simulink model "Candidacy_Exam_RR"  (R2023a)
settings: Solver=VariableStepAuto  StartTime=0  StopTime=1000  FixedStep=0.01  RelTol=1e-3
model workspace (MAT data in the model file):
  finalint = 0
  firstWarning = 1
  originalScenarioChecksum = '114339432DE22364D47BB28FC96DC10C'
undefined symbols (not defined in the file): Acceleration, ActorID, AngularVelocity, curvature, DefaultGear, Defined, DEND_B, DEND_S, DEND_T, direction, DiscIntNeverNeededParam, driving, Ego, EgoRefPose, gradbp, L, Lane, LF, LR, m, matlabshared, MAX_BRAKE, MAX_STEER, MAX_TORQUE, maxNumActors, MCAR, MIN_BRAKE, MIN_STEER, MIN_TORQUE, n, NUMD_B, NUMD_S, NUMD_T, Pitch, Pose, Position, psi_o, R, Roll, RRdamp, SceneInfo, session, sigbuilder_block, STEER_RATIO, stopSign_ID, Tdead, thetaRefs, TL_ID, TrackWidth, Ts, ts, User, Vdead, Velocity, WB, X_o, xRef2s, Y_o, Yaw, yRef2s
libraries: drivingscenarioandsensors x13, roadrunnerscenario x11, simulink x8, simulink_extras x5, drivingvehiclecontroller x2, trackingutilitieslib x2, robotalgslib x1, mpcadaslib x1, slpidlib x1, drivinglib x1, autolibshared x1, vehdynlibviscommon x1
(part 4 of 5)

== system Candidacy_Exam_RR/Reference Data1/Subsystem1/Subsystem3/Subsystem/Theta ==
  note: 1) Add Subsystem or Model blocks as valid variant choices.
      | 2) You cannot connect blocks at this level. At simulation, connectivity is automatically
      | determined, based on the active variant and port name matching.
  y : Inport
  x : Inport  Port=2
  dis : Inport  Port=3
  thetaBlocks : Subsystem  VariantControl=thetaSimulinkBlock
  thetaLt : Subsystem  VariantControl=thetaLookUpTable
  theta : Outport

== system Candidacy_Exam_RR/Reference Data1/Subsystem2/Subsystem/Theta/thetaBlocks ==
  note: theta calculated from Simulink blocks
  y : Inport
  x : Inport  Port=2
  dis : Inport  Port=3
  Atan2 : Trigonometry  Operator=atan2  ApproximationMethod=CORDIC
  Difference : simulink/Discrete/Difference  ICPrevInput=0.0  OutMin=[]  OutMax=[]  OutDataType=fixdt(1, 16)  OutScaling=2^-10  DoSatur=off
  Difference1 : simulink/Discrete/Difference  ICPrevInput=0.0  OutMin=[]  OutMax=[]  OutDataType=fixdt(1, 16)  OutScaling=2^-10  DoSatur=off
  IC : InitialCondition  Value=psi_o
  Radians to Degrees : simulink_extras/Transformations/Radians to Degrees
  Terminator : Terminator
  theta : Outport
  wires:
  IC/1 -> Radians to Degrees/1
  Atan2/1 -> IC/1
  dis/1 -> Terminator/1
  x/1 -> Difference1/1
  y/1 -> Difference/1
  Radians to Degrees/1 -> theta/1
  Difference/1 -> Atan2/1
  Difference1/1 -> Atan2/2

== system Candidacy_Exam_RR/Reference Data1/Subsystem2/Subsystem/Theta/thetaLt ==
  note: Check out the script "setUpModel" to understand how we have calculated theta
  note: theta based on lookup table
  y : Inport
  x : Inport  Port=2
  dis : Inport  Port=3
  Terminator : Terminator
  Terminator1 : Terminator
  Theta Ref : Lookup_n-D  NumberOfTableDimensions=1  BreakpointsForDimension1=gradbp  Table=thetaRefs  InternalRulePriority=Speed  RndMeth=Simplest
  theta : Outport
  wires:
  Theta Ref/1 -> theta/1
  dis/1 -> Theta Ref/1
  x/1 -> Terminator1/1
  y/1 -> Terminator/1

== system Candidacy_Exam_RR/Reference Data1/Subsystem3/Subsystem/Theta/thetaBlocks ==
  note: theta calculated from Simulink blocks
  y : Inport
  x : Inport  Port=2
  dis : Inport  Port=3
  Atan2 : Trigonometry  Operator=atan2  ApproximationMethod=CORDIC
  Difference : simulink/Discrete/Difference  ICPrevInput=0.0  OutMin=[]  OutMax=[]  OutDataType=fixdt(1, 16)  OutScaling=2^-10  DoSatur=off
  Difference1 : simulink/Discrete/Difference  ICPrevInput=0.0  OutMin=[]  OutMax=[]  OutDataType=fixdt(1, 16)  OutScaling=2^-10  DoSatur=off
  IC : InitialCondition  Value=psi_o
  Radians to Degrees : simulink_extras/Transformations/Radians to Degrees
  Terminator : Terminator
  theta : Outport
  wires:
  IC/1 -> Radians to Degrees/1
  Atan2/1 -> IC/1
  dis/1 -> Terminator/1
  x/1 -> Difference1/1
  y/1 -> Difference/1
  Radians to Degrees/1 -> theta/1
  Difference/1 -> Atan2/1
  Difference1/1 -> Atan2/2

== system Candidacy_Exam_RR/Reference Data1/Subsystem3/Subsystem/Theta/thetaLt ==
  note: Check out the script "setUpModel" to understand how we have calculated theta
  note: theta based on lookup table
  y : Inport
  x : Inport  Port=2
  dis : Inport  Port=3
  Terminator : Terminator
  Terminator1 : Terminator
  Theta Ref : Lookup_n-D  NumberOfTableDimensions=1  BreakpointsForDimension1=gradbp  Table=thetaRefs  InternalRulePriority=Speed  RndMeth=Simplest
  theta : Outport
  wires:
  Theta Ref/1 -> theta/1
  dis/1 -> Theta Ref/1
  x/1 -> Terminator1/1
  y/1 -> Terminator/1

== system Candidacy_Exam_RR/Reference Data1/Subsystem1/Subsystem2/Subsystem/Theta/thetaBlocks ==
  note: theta calculated from Simulink blocks
  y : Inport
  x : Inport  Port=2
  dis : Inport  Port=3
  Atan2 : Trigonometry  Operator=atan2  ApproximationMethod=CORDIC
  Difference : simulink/Discrete/Difference  ICPrevInput=0.0  OutMin=[]  OutMax=[]  OutDataType=fixdt(1, 16)  OutScaling=2^-10  DoSatur=off
  Difference1 : simulink/Discrete/Difference  ICPrevInput=0.0  OutMin=[]  OutMax=[]  OutDataType=fixdt(1, 16)  OutScaling=2^-10  DoSatur=off
  IC : InitialCondition  Value=psi_o
  Radians to Degrees : simulink_extras/Transformations/Radians to Degrees
  Terminator : Terminator
  theta : Outport
  wires:
  IC/1 -> Radians to Degrees/1
  Atan2/1 -> IC/1
  dis/1 -> Terminator/1
  x/1 -> Difference1/1
  y/1 -> Difference/1
  Radians to Degrees/1 -> theta/1
  Difference/1 -> Atan2/1
  Difference1/1 -> Atan2/2

== system Candidacy_Exam_RR/Reference Data1/Subsystem1/Subsystem2/Subsystem/Theta/thetaLt ==
  note: Check out the script "setUpModel" to understand how we have calculated theta
  note: theta based on lookup table
  y : Inport
  x : Inport  Port=2
  dis : Inport  Port=3
  Terminator : Terminator
  Terminator1 : Terminator
  Theta Ref : Lookup_n-D  NumberOfTableDimensions=1  BreakpointsForDimension1=gradbp  Table=thetaRefs  InternalRulePriority=Speed  RndMeth=Simplest
  theta : Outport
  wires:
  Theta Ref/1 -> theta/1
  dis/1 -> Theta Ref/1
  x/1 -> Terminator1/1
  y/1 -> Terminator/1

== system Candidacy_Exam_RR/Reference Data1/Subsystem1/Subsystem3/Subsystem/Theta/thetaBlocks ==
  note: theta calculated from Simulink blocks
  y : Inport
  x : Inport  Port=2
  dis : Inport  Port=3
  Atan2 : Trigonometry  Operator=atan2  ApproximationMethod=CORDIC
  Difference : simulink/Discrete/Difference  ICPrevInput=0.0  OutMin=[]  OutMax=[]  OutDataType=fixdt(1, 16)  OutScaling=2^-10  DoSatur=off
  Difference1 : simulink/Discrete/Difference  ICPrevInput=0.0  OutMin=[]  OutMax=[]  OutDataType=fixdt(1, 16)  OutScaling=2^-10  DoSatur=off
  IC : InitialCondition  Value=psi_o
  Radians to Degrees : simulink_extras/Transformations/Radians to Degrees
  Terminator : Terminator
  theta : Outport
  wires:
  IC/1 -> Radians to Degrees/1
  Atan2/1 -> IC/1
  dis/1 -> Terminator/1
  x/1 -> Difference1/1
  y/1 -> Difference/1
  Radians to Degrees/1 -> theta/1
  Difference/1 -> Atan2/1
  Difference1/1 -> Atan2/2

== system Candidacy_Exam_RR/Reference Data1/Subsystem1/Subsystem3/Subsystem/Theta/thetaLt ==
  note: Check out the script "setUpModel" to understand how we have calculated theta
  note: theta based on lookup table
  y : Inport
  x : Inport  Port=2
  dis : Inport  Port=3
  Terminator : Terminator
  Terminator1 : Terminator
  Theta Ref : Lookup_n-D  NumberOfTableDimensions=1  BreakpointsForDimension1=gradbp  Table=thetaRefs  InternalRulePriority=Speed  RndMeth=Simplest
  theta : Outport
  wires:
  Theta Ref/1 -> theta/1
  dis/1 -> Theta Ref/1
  x/1 -> Terminator1/1
  y/1 -> Terminator/1

== matlab function Candidacy_Exam_RR/Controllers/Longitudinal Controllers/Velocity Profiler ==
  data: distanceToScene input; referenceVelocity output; BrakingPhase output; slowDownFlag input; safeStopDistance input; CurrVel input; desiredVelocity input; distTravelled input; X_f input; a_coeff input; X_f output; a_coeff output
function [referenceVelocity, BrakingPhase, X_f, a_coeff]   = VelocityProfiler(distanceToScene, slowDownFlag, safeStopDistance, CurrVel, desiredVelocity, distTravelled, X_f, a_coeff)

% if ~brakingFlag     
%     referenceVelocity = desiredVelocity;
% else
%     if DesiredDecel == 0
%         DesiredDecel = (CurrVel^2)/(2*dist);
%         referenceVelocity = sqrt(2*dist*DesiredDecel);
%     else
%         referenceVelocity = sqrt(2*max(dist - safeStopDistance, 0)*DesiredDecel);
%     end
% end
% 
% end
BrakingPhase = 0;
D2S = abs(distanceToScene);
xx = 5;
vel = 1;
if ~slowDownFlag
    referenceVelocity = desiredVelocity;
    X_f = 0; 
elseif slowDownFlag && X_f == 0
    X_i = 0;
    X_f = D2S - xx; % Initial D2S at the moment when flag is raised (velocity poly starts from zero)

    P = [1, X_i, X_i^2, X_i^3, X_i^4, X_i^5;
         0, 1, 2*X_i, 3*X_i^2, 4*X_i^3, 5*X_i^4;
         0, 0, 2, 6*X_i, 12*X_i^2, 20*X_i^3;
         1, X_f, X_f^2, X_f^3, X_f^4, X_f^5;
         0, 1, 2*X_f, 3*X_f^2, 4*X_f^3, 5*X_f^4;
         0, 0, 2, 6*X_f, 12*X_f^2, 20*X_f^3];

    % Initial Conditions
    Vx_i = CurrVel; 
    Ax_i = 0; 
    Vx_f = vel;
    Ax_f = -0.5; 
    Jx_i = 0;
    Jx_f = 0;
    InitialCond = [Vx_i; Ax_i; Jx_i; Vx_f; Ax_f; Jx_f];
    a_coeff = P\InitialCond;
    distCovered  = abs(X_f - (D2S - xx));
    referenceVelocity = max([1,distCovered,distCovered^2,distCovered^3,distCovered^4,distCovered^5]*a_coeff, 0);
else
    distCovered  = abs(X_f - (D2S - xx));
    if D2S <= 2.5 % distCovered >= (X_f + 4)
        referenceVelocity = 0;
        BrakingPhase = 3;
    elseif D2S <= xx % distCovered >= X_f
        referenceVelocity = vel;
        BrakingPhase = 2;
    else
        BrakingPhase = 1;
        referenceVelocity = max([1,distCovered,distCovered^2,distCovered^3,distCovered^4,distCovered^5]*a_coeff, 0);
    end

end

end

== matlab function Candidacy_Exam_RR/Controllers/Longitudinal Controllers/Subsystem/Velocity - Curvature ==
  data: desiredVelocity input; referenceVelocity output; curveMinThreshold input; curvature input
function referenceVelocity = velocityCurveCalculation(desiredVelocity,curveMinThreshold, curvature)

    if abs(curvature) >= 0 && abs(curvature) <= curveMinThreshold
        referenceVelocity = desiredVelocity;
    else
        r = 1/abs(curvature);
        referenceVelocity = min(desiredVelocity, sqrt(9.81*r*0.9*0.4));
    end

== matlab function Candidacy_Exam_RR/Controllers/Longitudinal Controllers/Subsystem/Curvature Calculation ==
  data: RefXY input; curvatureAhead output; SlowdownDistance input; minimumCurvatureThreshold input; cumulativeDistance output
function [curvatureAhead, cumulativeDistance] = CurvatureCalculation(RefXY, SlowdownDistance, minimumCurvatureThreshold)

% minimumCurvatureThreshold: curvature value above which it is considered
% straight, not curved path

DX = gradient(RefXY(:, 1));
D2X = gradient(DX);
DY = gradient(RefXY(:,2));
D2Y = gradient(DY);
curvature = (DX.*D2Y - DY.*D2X) ./(DX.^2+DY.^2).^(3/2);

% Calculate Distance Vector
distanceMatrix = squareform(pdist(RefXY));
distanceSteps = zeros(length(RefXY)-1,1);
for i = 2:length(RefXY)
    distanceSteps(i-1,1) = distanceMatrix(i,i-1);
end
totalDistance = sum(distanceSteps); % Total distance travelled along reference path
cumulativeDistance = cumsum([0; distanceSteps]); % Distance for each waypoint

% Curvature Ahead Calculation
st = 0;
en = 1;
j1 = 1;
CurveInfo = zeros(length(curvature),7); % [startX startY endX endY MaxCurve startidx endidx]

for j = 1:length(curvature)
    if abs(curvature(j)) >= minimumCurvatureThreshold
        if abs(curvature(j)) >= CurveInfo(j1,5)
            CurveInfo(j1,5) = abs(curvature(j));
        end
        if st == 0
            CurveInfo(j1,1:2) = [RefXY(j,1) RefXY(j,2)]; % Startpoint
            CurveInfo(j1,6) = j;
            st = 1;
            en = 0;
        end
    elseif (abs(curvature(j)) < minimumCurvatureThreshold) && (en == 0)
            CurveInfo(j1,3:4) = [RefXY(j,1) RefXY(j,2)]; % Endpoint
            CurveInfo(j1,7) = j;
            j1 = j1+1;
            st = 0;
            en = 1;
    end
    if (j == length(curvature)) && (en == 0)
           CurveInfo(j1,3:4) = [RefXY(j,1) RefXY(j,2)]; % Endpoint
            CurveInfo(j1,7) = j;
            j1 = j1+1;
            st = 0;
            en = 1;
    end
end

j2 = 1;
curvatureAhead = zeros(length(curvature),1);
if j1 > 1
    for j = 1:length(cumulativeDistance)
        if (cumulativeDistance(j) >= (cumulativeDistance(CurveInfo(j2, 6)) - SlowdownDistance)) && (cumulativeDistance(j) < cumulativeDistance(CurveInfo(j2,7)))
            curvatureAhead(j) = CurveInfo(j2,5);
        elseif (cumulativeDistance(j) >= cumulativeDistance(CurveInfo(j2,7))) && (j2 < j1-1)
            curvatureAhead(j) = CurveInfo(j2,5);
            j2 = j2+1;
        else
            curvatureAhead(j) = curvature(j);
        end
    end
end

== matlab function Candidacy_Exam_RR/Controllers/Longitudinal Controllers/Subsystem/Reference Pose Search ==
  data: RefXY input; currentPose input; referenceCurvature input; curvature output; cumulativeDistance input; currentDistanceTravelled output
function [curvature, currentDistanceTravelled] = referencePoseSearch(RefXY, currentPose, referenceCurvature, cumulativeDistance)

dist = zeros(length(RefXY),1);
for j = 1:length(RefXY)
    dist(j) = norm(currentPose(1:2) - RefXY(j,1:2));
end

[~, ind] = mink(dist,2);

if ind(1) > ind(2)
    ind = [ind(2); ind(1)];
end

curvature = referenceCurvature(ind(1));
currentDistanceTravelled = cumulativeDistance(ind(1)) + norm(RefXY(ind(1),1:2) - currentPose(1:2));


% referencePoses = zeros(1, 2);
% m = 0; mm = 0; b = 0; bb = 0;
% m = (RefXY(ind(1),2) - RefXY(ind(2),2))/(RefXY(ind(1),1) - RefXY(ind(2),1));
% if m == inf
%     referencePoses = [RefXY(ind(1),1) currentPose(2)];
% elseif m == 0
%     referencePoses = [currentPose(1) RefXY(ind(1),2)];
% else
%     b = RefXY(ind(1),2) - m*RefXY(ind(1),1);
%     mm = -1/m;
%     bb = currentPose(2) - mm*currentPose(1);
%     referencePoses(1:2) = [(b-bb)/(mm-m) m*((b-bb)/(mm-m)) + b];
% 
% end
% positionError = norm(referencePoses(1:2) - currentPose(1:2));

== matlab function Candidacy_Exam_RR/Environment & Data/Roadrunner Port/MATLAB Function1 ==
  data: u input; long_out output; lat_out output; z_out output; out output; final_x output; final_y output
function [long_out, lat_out, z_out, out, final_x, final_y]  = fcn(u)
out = zeros(500, 3);
long = zeros(500, 1);
lat = zeros(500, 1);
long = u(:, 2);
lat = u(:,1);

for i = 1:500
    if long(i) == 0 && lat(i) == 0
        long(i) = long(i-1); 
        lat(i) = lat(i-1);
    end
end
final_x = lat(end);
final_y = long(end);
out(:,1) = lat;
out(:,2) = long;
out(:,3) = u(:, 3);

lat_out = out(:,1);
long_out = out(:, 2);
z_out =  out(:, 3);

== matlab function Candidacy_Exam_RR/Controllers/Subsystem2/MATLAB Function ==
  data: u input; accel output; decel output
function [accel, decel] = fcn(u)
if(u>0)
    accel=u; decel=0;
elseif(u<0)
    accel=0; decel=-u;
else
    accel=0;decel=0;
end

== matlab function Candidacy_Exam_RR/Controllers/Subsystem2/Subsystem/Desired Velocity Profile ==
  data: MaxBrakeFlag output; CurrVel input; DesiredDecel output; RelDist input; Dist1 output; StoppingDist input
function [MaxBrakeFlag,DesiredDecel,Dist1] = VelocityProfile(CurrVel,RelDist,StoppingDist)
% time remaining = (current velocity) / (deceleration).
% desired velocity = (stopping distance - current distance) / time remaining.
Dist1 = RelDist - (2.6850+1);
Dist = Dist1 - StoppingDist;
if Dist1 <= 2
    MaxBrakeFlag = 1;
    DesiredDecel = 0;
else
    MaxBrakeFlag = 0;
    DesiredDecel = min((CurrVel^2)/(2*Dist),3);
end
%     Dist = RelDist - (2.6850 + 3);
%     Decel = (CurrVel^2)/(2*Dist);
%     RemainingTime = CurrVel/Decel;
%     DesiredVel = Dist/RemainingTime; % DesiredVel = CurrVel/2

== matlab function Candidacy_Exam_RR/Controllers/Subsystem2/Subsystem/Function-Call Subsystem/MATLAB Function1 ==
  data: Vel input; BrakingAcc output; RelDist input
function BrakingAcc = fcn(Vel,RelDist)

DistOffset = 1;
Dist = RelDist - DistOffset;
BrakingAcc = (Vel^2)/(2*Dist);

== matlab function Candidacy_Exam_RR/Environment & Data/Roadrunner Port/Pack Actor Pose/Pose Generation ==
  data: pose input; currPose output
function currPose = generatePose(pose)

yaw = deg2rad(pose(3));
rotm = eul2rotm([yaw 0 0]);

currPose = [[rotm [pose(1:2) 0]']; [0 0 0 1]];
% currPose = [[rotm [pose(1:2) 235]']; [0 0 0 1]];

== matlab function Candidacy_Exam_RR/Environment & Data/Roadrunner Port/Pack Actor Pose/Velocity XYZ Components ==
  data: yaw input size=1; velocity output size=[1 3]; speed input size=1
function velocity = computeVelocity(yaw, speed)

% Output velocity vector (x,y,z)
velocity = speed * [-sind(yaw) cosd(yaw) 0];

== matlab function Candidacy_Exam_RR/Vehicle Dynamics/VehicleDynamics/MATLAB Function ==
  data: InitialPos input; Xo output; Yo output
function [Xo, Yo] = fcn(InitialPos)

Xo = InitialPos(1);
Yo = InitialPos(2);

== matlab function Candidacy_Exam_RR/Controllers/Longitudinal Controllers/MATLAB Function1 ==
  settings: updateMethod=DISCRETE
  data: u input; y output
function y = fcn(u)
persistent flag cnt
t = 200;
if isempty(cnt)
        cnt = 0;
end
if isempty(flag)
        flag = 0;
end
    if u == 0
        flag = 1;
        y = 0;
    elseif u == 1 && flag == 1
        y = 1;
        cnt = cnt + 1;
        if cnt > t
            cnt = 0;
            flag = 0;
        end

    elseif u == 2 && flag == 0
        cnt = cnt + 1;
        if cnt > t
            cnt = 0;
            flag = 1;
        end
        y = 1;
    elseif u == 3 && flag == 1
        cnt = cnt + 1;
        if cnt > t
            cnt = 0;
            flag = 0;
        end
        y = 1;
    else
        y = 0;
    end

end

== matlab function Candidacy_Exam_RR/Environment & Data/Visualisation & Data/Positions and States /MATLAB Function2 ==
  data: Actors input; ss_poses output; ss_State input

function ss_poses = findssposes(Actors, ss_State)

n=length(ss_State);
ss_poses=zeros(n,4);
indices=zeros(n,1);
ID=zeros(length(Actors),1);

for i=1:length(Actors)
 ID(i)=Actors(i).ActorID;
end

indices=find(ismember(ID,ss_State));
if(~isempty(indices))
    
    for i=1:n
        ss_poses(i,:)=([Actors(indices(i)).Position(:)',ss_State(i)]);
    end
end

ss_poses(ss_poses==0)=NaN;






% ss1_poses=zeros(1,4);
% ss2_poses=zeros(1,4);
% for i=1:length(Actors)
%     ID=Actors(i).ActorID;
%     
%     if(ID==ss1_State(1))
%         ss1_poses=[Actors(i).Position(:)',ss1_State(1)];
%     elseif ID== (ss1_State(2))
%         ss2_poses=[Actors(i).Position(:)',ss1_State(2)];
%     
%     end
%   
% end
% ss1_poses(ss1_poses==0)=NaN;   
% ss2_poses(ss2_poses==0)=NaN;

== matlab function Candidacy_Exam_RR/Environment & Data/Visualisation & Data/Positions and States /MATLAB Function1 ==
  data: Actors input; TL_poses output; TL_State input

function TL_poses = findTLposes(Actors, TL_State)
n=length(TL_State);
TL_poses=zeros(n/2,5);
indices=zeros(n/2,1);
ID=zeros(length(Actors),1);

for i=1:length(Actors)
 ID(i)=Actors(i).ActorID;
end

indices=find(ismember(ID,TL_State(n/2+1:end)));
if (~isempty(indices))

    for i=1:n/2
        TL_poses(i,:)=([Actors(indices(i)).Position(:)',TL_State(i),ID(indices(i))]);

    end
end
TL_poses(TL_poses==0)=NaN;

== stateflow chart Candidacy_Exam_RR/Environment & Data/Visualisation & Data/Positions and States /Traffic Light Sensor/Traffic Light Switching Logic ==
  state STEADYRED
    entry:
    trafficLight(:)= Red; TL_ID=TL_id;
  state STEADYGREEN
    entry:
    trafficLight(:)= Green; TL_ID=TL_id;
  state START
    entry:
    trafficLight=TL_id;
    trafficLight(:)= Black;TL_ID=TL_id;
  state TRAFFICLIGHT_ODDYELLOW_EVENRED
    entry:
    trafficLight(1:2:end)=Yellow;TL_ID(1:2:end)=TL_id(1:2:end);
    trafficLight(2:2:end) = Red;TL_ID(2:2:end)=TL_id(2:2:end);
  state TRAFFICLIGHT_ODDGREEN_EVENRED
    entry:
    trafficLight(1:2:end)=Green;TL_ID(1:2:end)=TL_id(1:2:end);
    trafficLight(2:2:end) = Red;TL_ID(2:2:end)=TL_id(2:2:end);
  state TRAFFICLIGHT_ODDRED_EVENYELLOW
    entry:
    trafficLight(1:2:end)=Red;TL_ID(1:2:end)=TL_id(1:2:end);
    trafficLight(2:2:end) = Yellow;TL_ID(2:2:end)=TL_id(2:2:end);
  state TRAFFICLIGHT_ODDRED_EVENGREEN
    entry:
    trafficLight(1:2:end)=Red;TL_ID(1:2:end)=TL_id(1:2:end);
    trafficLight(2:2:end) = Green;TL_ID(2:2:end)=TL_id(2:2:end);
  (default) -> START
  START -> STEADYGREEN [order 3] : [LightConfig==1]
  START -> STEADYRED [order 1] : [LightConfig==2]
  START -> TRAFFICLIGHT_ODDGREEN_EVENRED [order 2] : [LightConfig ==3]
  TRAFFICLIGHT_ODDGREEN_EVENRED -> TRAFFICLIGHT_ODDYELLOW_EVENRED : after(4,sec)
  TRAFFICLIGHT_ODDYELLOW_EVENRED -> TRAFFICLIGHT_ODDRED_EVENGREEN : after(1,sec)
  TRAFFICLIGHT_ODDRED_EVENYELLOW -> TRAFFICLIGHT_ODDGREEN_EVENRED : after(1,sec)
  TRAFFICLIGHT_ODDRED_EVENGREEN -> TRAFFICLIGHT_ODDRED_EVENYELLOW : after(4,sec)
  data: Green constant double =3; Red constant double =1; Yellow constant double =2; LightConfig input; TL_id input; Black constant double =0; TL_ID output; trafficLight output

== matlab function Candidacy_Exam_RR/Environment & Data/Sensors & Perception/MATLAB Function ==
  data: SceneID output; ObjRelVel output; SceneRelVel output; SceneDist output; ObjectDist output; ObjAhead output; SDist input; Tracking input; SceneAhead output; RelVelmin output; RelDistmin output; Trans input; ObjectMIO_Position output; ObjTracks output; SceneTracks output
function [SceneID,ObjRelVel,SceneRelVel,SceneDist,ObjectDist,ObjAhead,SceneAhead,RelVelmin,RelDistmin,ObjectMIO_Position,ObjTracks,SceneTracks]= SFDetections(SDist,Tracking, Trans)
ObjectID = zeros(20,1);
TrackPos = zeros(3,20);
TrackVel = zeros(3,20);
ObjTracks = zeros(6,20);
SceneTracks = zeros(6,20);
ObjectDist = 100; % zeros(20,1);
SceneDist = 100;
ObjRelVel = 10;
SceneRelVel = 10;
% ScenePos = [0 0];
ObjAhead = 0;
SceneAhead = 0;
SceneID = 0;
% TracksNum = Tracking.NumTracks;
TracksNum = 0;
ObjectMIO_Position = zeros(3,1);
s1 = 0;
s2 = 0;

% Tracks from sensors
% TracksNum = Tracking.NumTracks;

% Ground truth
TracksNum1 = Tracking.NumActors;
% reading only tracks in the field of view (180 deg)
for k = 1:TracksNum1
    ang = atan2d(Tracking.Actors(k).Position(2),Tracking.Actors(k).Position(1));
    if abs(ang) < 90
        TracksNum = TracksNum + 1;
        ObjectID(TracksNum) = Tracking.Actors(k).ActorID;
        TrackPos(:,TracksNum) = Tracking.Actors(k).Position;
        TrackVel(:,TracksNum) = Tracking.Actors(k).Velocity;
    end
end

for t = 1:TracksNum
    % ObjectID(t) = Tracking.Tracks(t).ObjectClassID;
    % TrackPos(:,t) = Tracking.Tracks(t).State(1:2:5);
    % TrackVel(:,t) = Tracking.Tracks(t).State(2:2:6);

    % All objects and scene Detections
    

    if ObjectID(t) == 7 % Scenes: 7=SS 8=TL 9=RA 10=RRC % labels {1,2,3,4} => {'TrafficLight','StopSign','RailRoadCrossing','RoundAbout'};
        s1 = s1 + 1;
        % Tracks from sensors
        % SceneTracks(:,s1) = Tracking.Tracks(t).State(:);

        % Ground Truth
        SceneTracks(:,s1) = [TrackPos(1,t) TrackVel(1,t) TrackPos(2,t) TrackVel(2,t) TrackPos(3,t) TrackVel(3,t)]';
    elseif ObjectID(t) < 7 && ObjectID(t) > 0 % Objects
        s2 = s2 + 1;
        % Tracks from sensors
        % ObjTracks(:,s2) = Tracking.Tracks(t).State(:);

        % Ground Truth
        ObjTracks(:,s2) = [TrackPos(1,t) TrackVel(1,t) TrackPos(2,t) TrackVel(2,t) TrackPos(3,t) TrackVel(3,t)]';
    end
   




    if TrackPos(2,t) < 1 && TrackPos(2,t) > -10 && abs(TrackPos(1,t)) <= SDist
        
        if ObjectID(t) >= 7  && Trans ~= 1% 7=SS 8=TL 9=RA 10=RRC % labels {1,2,3,4} => {'TrafficLight','StopSign','RailRoadCrossing','RoundAbout'};
            SceneAhead = 1;
            SceneDist = min(SceneDist,TrackPos(1,t));
            if TrackPos(1,t) <= SceneDist
                % ScenePos = TrackPos(1:2,t)';
                SceneRelVel = TrackVel(1,t);
                SceneID = ObjectID(t);
            end
        end

        if ObjectID(t) < 7 && ObjectID(t) > 0
            ObjAhead = 1;
            ObjectDist = min(ObjectDist,TrackPos(1,t));
            ObjectMIO_Position(:,1) = TrackPos(:,t);

            if TrackPos(1,t) <= ObjectDist
                ObjRelVel = TrackVel(1,t);
                ObjID = ObjectID(t);
            end
        end

    end
    
end

if Trans == 1  % ObjectDist <= SceneDist
    RelVelmin = ObjRelVel;
    RelDistmin = ObjectDist;
else
    RelVelmin = min(SceneRelVel,ObjRelVel);
    RelDistmin = min(SceneDist,ObjectDist);
end

== matlab function Candidacy_Exam_RR/Vehicle Dynamics/Info2ActorState/MATLAB Function ==
  data: X input; Position output; Y input; Z input
function Position = fcn(X, Y, Z)

Position = [X Y, Z];

== matlab function Candidacy_Exam_RR/Subsystem/PathPlanner/MATLAB Function4 ==
  data: Distance output; output input; CurrentPose input; point output
function [Distance,point] = d2f(output,CurrentPose)



%Distance = norm(output(end,:) - CurrentPose(1:2)');
Distance= output(end,1)- CurrentPose(1);
point=output(end,:);

end

%Distance = sqrt(CurrentPose(1)-output(99,1))^2 + (CurrentPose(2)-output(99,2)^2);
%CurrentPose
%output=zeros(99,2);
%lastPoint = output(end,:);
%dx = lastPoint(1) - x;
%dx= output(end,1)-x;
%dy = output(end,2) - y;
%distance = sqrt(dx^2 + dy^2);

== matlab function Candidacy_Exam_RR/Environment & Data/Sensors & Perception/MATLAB Function1 ==
  data: EVpos input; yaw input; SceneID input; SceneInfo input; SDir output; SDist input; D2S output
function [SDir,D2S] = SceneFinder(EVpos,yaw, SceneID, SceneInfo, SDist)
D2S = zeros(10,1);
    % dist = zeros(1,length(SceneLocations));
    for j = 1:length(SceneInfo(:,1))
        distXY = SceneInfo(j,1:2) - EVpos(1:2);
        D2S(j) = norm(distXY);
        
%         if (D2S <= SDist)
%             Scene = SceneInfo(j,3); % labels {1,2,3,4} => {'TrafficLight','StopSign','RailRoadCrossing','RoundAbout'};
%             angl = atan2d(distXY(2),distXY(1));
%             angl = angl - yaw;
% %             rot = [cosd(angl) -sind(angl);sind(angl) cosd(angl)];
% %             distXY = rot*distXY';
% %             angl = atan2d(distXY(2),distXY(1));
%             
%             if angl < 0
%                 angl = angl + 360;
%             end
% 
%             if (angl > 315) || (angl <= 45) 
%                 SDir = "N";
%             elseif (angl > 225) && (angl <= 315)
%                 SDir = "E";
%             elseif (angl > 135) && (angl <= 225)
%                 SDir = "S";
%                 D2S = 1000;
%                 angl = 1000;
%                 Scene = 0;
%             elseif (angl > 45) && (angl <= 135)
%                 SDir = "W";
%             else
%                 SDir = "Error";
%             end
%             break
%         else
%             Scene = 0;
%             SDir = " ";
%             angl = 1000;
%             D2S = 1000;
%         end

    end
[val,indx] = min(D2S);

== matlab function Candidacy_Exam_RR/Subsystem/Function-Call Subsystem/MATLAB Function2 ==
  data: EgoPosition input; MIOPos input; curvature input; MIOVel input; V_i input; xd output; yd output; laneL input; laneR input; V_desired input; LCinProgress output
function [xd,yd,LCinProgress] = traj(EgoPosition,MIOPos,curvature,MIOVel, V_i, laneL, laneR, V_desired)
Vx_i =0;Vx_f=0;Vy_i=0;Vy_f=0;Ax_i=0;Ax_f=0;Ay_i=0;Ay_f=0;T_i=0;T_f=0;V_f=0;A_f=0;x_set=0;y_set=0;theta4=0;

P = zeros(6,6);
% xq = zeros(1,size(RefPath,1)); yq = zeros(1,size(RefPath,2));
EgoPosition(1,2)=-EgoPosition(1,2)
x_init= EgoPosition(1,1)+0.5; y_init = EgoPosition(1,2)-0.8;
% xq = RefPath(:,1)'; 
% yq = RefPath(:,2)';
num_foc_t = 98;
V_max= V_desired; ad_n=0; vd_n=MIOVel; wd_n=vd_n*curvature;
lane_width = 3.6 * (laneL-laneR); % +1 if left of current lane and -1 if right of current lane
xd = zeros(num_foc_t+1,1); 
yd = zeros(num_foc_t+1,1);
xf =0; 
yf = 0;

    %xf = [EgoPosition(1,1)+ MIOPos(1) ]; yf = [ EgoPosition(1,2)+ MIOPos(2) + lane_width];  
    xf = [EgoPosition(1,1)+ 40 ]; yf = [ EgoPosition(1,2)+ 1.1*lane_width]; % 80
    V_f = V_max;
    W_f = V_f*curvature;
    A_f = 0;

    %dist2crash = sqrt((x_init-MIOPos(1))^2+(y_init-MIOPos(2))^2);
    %dist2crash = 40;
    %T_f = abs(dist2crash/(MIOVel-V_i));
    T_f = 3;
    P = [1, T_i, T_i^2, T_i^3, T_i^4, T_i^5;
         0, 1, 2*T_i, 3*T_i^2, 4*T_i^3, 5*T_i^4;
         0, 0, 2, 6*T_i, 12*T_i^2, 20*T_i^3;
         1, T_f, T_f^2, T_f^3, T_f^4, T_f^5;
         0, 1, 2*T_f, 3*T_f^2, 4*T_f^3, 5*T_f^4;
         0, 0, 2, 6*T_f, 12*T_f^2, 20*T_f^3];

%     mtang4 = (yq(1,index+2)-yq(1,index+1))/(xq(1,index+2)-xq(1,index+1));

    Vx_i = vd_n*cos(theta4); 
    Vy_i = vd_n*sin(theta4); 
    Ax_i = ad_n*cos(theta4)-vd_n*sin(theta4)*wd_n; 
    Ay_i = ad_n*sin(theta4)+vd_n*cos(theta4)*wd_n;

%     if(xq(index+2)-xq(index+1)<0)
%         theta_4 = pi + atan(mtang4);
%     else
%         theta_4 = atan(mtang4);
%     end

    theta_4 =0;
    Vx_f = V_f*cos(theta_4); % curvature angle
    Vy_f = V_f*sin(theta_4);
    Ax_f = A_f*cos(theta_4)-V_f*sin(theta_4)*W_f;
    Ay_f = A_f*sin(theta_4)+V_f*cos(theta_4)*W_f;

    g1 = [x_init; Vx_i; Ax_i; xf; Vx_f; Ax_f];
    g2 = [y_init; Vy_i; Ay_i; yf; Vy_f; Ay_f];

    a_coeff = P\g1;
    b_coeff = P\g2;
    
    td = T_i;
    scatter(x_init,y_init,'go')
    hold on; 
    scatter(xf,yf,'ro')
    hold on;
    
    for f = 1:(num_foc_t+1)
        xd(f,1) = [1,td,td^2,td^3,td^4,td^5]*a_coeff 
        yd(f,1) = [1,td,td^2,td^3,td^4,td^5]*b_coeff
        td = td + (T_f - T_i)/num_foc_t;
        scatter(xd(f,1),yd(f,1),'y.');
    end

LCinProgress = 1;

% hold on;
end

== stateflow chart Candidacy_Exam_RR/Behavioural Planner/Collision Avoidance ==
  state Stop
    en:
    HoldBrake = 1;
  state Start
    en:
    Stuck = 0;
    ACC = 0;
    LaneChangeCmd = 0;
    %VelCmd = CurrentVelCmd;
  state Follow
    en:
    ACC = 0;
    Brake = 1;
  state LaneChange
    en:
    LaneChangeCmd = 1;
    ACC=0;
  Stop -> Follow [commented out] : [EgoSpeed<0.1]
  Follow -> Stop [order 4] : [D2O < 5]
  Follow -> Stop [commented out] : [D2O < 5 && EgoSpeed > 2]
  (default) -> Start
  Follow -> LaneChange [order 2] : [LC_ACC==1]
  Start -> Follow : [ObjAhead == 1]
  Follow -> Start [order 3] : [ObjAhead == 0]
  LaneChange -> Start : [LaneChanged == 1]
  Follow -> Follow [order 1] : [(EgoSpeed <= MinSpeed) && after(WaitTime,sec)]{Stuck = 1;}
  data: Stuck local; ACC output; WaitTime input; ObjAhead input; MinSpeed input; LaneAvailable input; EgoSpeed input; LaneChanged input; LC_ACC input; LaneChangeCmd output; Brake output; D2O input; HoldBrake output

== matlab function Candidacy_Exam_RR/Behavioural Planner/Destination ==
  data: u input; y output
function y = fcn(u)

y = [u(end,1) u(end,2)];
end

== matlab function Candidacy_Exam_RR/Controllers/MATLAB Function2 ==
  data: v input; RefVelCmd output; curvature input
function RefVelCmd = fcn(v,curvature)

    if abs(curvature) >= 0 && abs(curvature) <= 2e-2
        RefVelCmd = v;
    else
        r = 1/abs(curvature);
        RefVelCmd = min(v,sqrt(9.81*r*.2));
    end

== matlab function Candidacy_Exam_RR/Vehicle Dynamics/Info2ActorState/MATLAB Function1 ==
  data: Xdot input; Velocity output; Ydot input; Zdot input
function Velocity = fcn(Xdot, Ydot, Zdot)

Velocity = [Xdot Ydot, Zdot];

== stateflow chart Candidacy_Exam_RR/Behavioural Planner/Emergency Stop ==
  state EmergencyCheck
    en:
    EStop = 0;
  state Pullover
    en:
    EStop=1;
  state Stop
    en:
    EStop=2;
  Pullover -> EmergencyCheck : [TechFailure == 0]
  (default) -> EmergencyCheck
  EmergencyCheck -> Pullover [order 1] : [TechFailure == 1]
  EmergencyCheck -> Stop [order 2] : [D2O<=1]
  Stop -> EmergencyCheck : [D2O > 2]
  data: D2O input; TechFailure input; EStop output

== matlab function Candidacy_Exam_RR/MATLAB Function ==
  data: ttc output; dist output; left output; right output; LL_avail output; RL_avail output; tend2stay output; ego input; act input; LaneBounds input; RoadSpeed input; ego_vel output; stay output; LL_Change output; RL_Change output; y_lane output; LCinProgress input
function [ttc,dist,left,right,LL_avail,RL_avail,tend2stay,ego_vel,stay,LL_Change,RL_Change,y_lane] = fcn(ego,act,LaneBounds,RoadSpeed, LCinProgress)                       


%% Major tasks to look into

% Check the performance while transitioning into another lane 
% Lane change output when the ego on extreme lanes.
% Develop code to handle lane changes on road curvatures
% Integrate with the trajectory generation and check the perfomance
% Convert the code to ego vehicle coordinates


%%
%define some parameters
r_c = 20; %range considered to MIOs
t_min =  2;

num_actors = length(act.Actors);
%num_lanes = length(LaneBounds.LaneBoundaries)-1;


%% Using sensor data 
% TracksNum = Tracking.NumTracks;
% 
% 
% for t = 1:TracksNum
%     ObjectID(t) = Tracking.Tracks(t).ObjectClassID;
%     TrackPos(:,t) = Tracking.Tracks(t).State(1:2:5);
%     TrackVel(:,t) = Tracking.Tracks(t).State(2:2:6);

%% ego position and  velocity magnitude
ego_pos = ego.Position;
ego_vel = ego.Velocity(1);  % velocity

%ttc: (array) : agent.relative position / abs(relative velocity)
ttc = zeros(1,num_actors);
left = zeros(1,num_actors);
right = zeros(1,num_actors);

dist =  zeros(1,num_actors);
tend2stay=1;

%%
y_lane = zeros(1,length(LaneBounds.LaneBoundaries))

for l=1:length(y_lane)
    y_lane(l)=LaneBounds.LaneBoundaries(l).Coordinates(end,2)
end

%%
for i= 1:num_actors

    % Grab actor positions and velocities
    actor_pos = act.Actors(i).Position;   
    actor_vel = act.Actors(i).Velocity(1);  % x-component velocity

    %relative velocity of the agent
    rel_vel = actor_vel - ego_vel;


    %% Check if the actor is within a r_c range. If it is out of range, pass lane change as '1' automatically.

   dist(i) = norm([actor_pos(1) actor_pos(2)]-[ego_pos(1) ego_pos(2)]);
        
    if dist(i) > r_c
        left(i)=1;
        right(i)=1;
        continue
    end

    %% Check if the actor is in the same lane as that of ego

    % If the actor and ego are in the same lane, it is considered a lead/following vehicle in the same lane and by defualt, the lane change flag is 1.

    if (actor_pos(2)< (ego_pos(2)+0.5) && actor_pos(2) > (ego_pos(2)-0.5))
        if (rel_vel < 0 && ego_vel < (RoadSpeed+5) && actor_pos(1) > ego_pos(1) )
            left(i) =1;
            right(i)=1;
            tend2stay=0;        % we need to incorporate too slow condition even when the relative velocity is greater than 0.

        elseif (rel_vel < 0 && ego_vel < (RoadSpeed+5) && actor_pos(1) < ego_pos(1) )
            left(i) =1;
            right(i)=1;
            tend2stay=1;
        end

        continue
    end

    
    %% calculate ttc for the rest of the vehicles


    ttc(i) = (actor_pos(1)-ego_pos(1))/abs(rel_vel);

    % checking conditions for other surrounding actors

    % all actors on the left lane of the ego vehicle
%%
    if actor_pos(2)-ego_pos(2) > 0  

        if and(rel_vel>0, ttc(i) > t_min)  % target vehicles on the front of ego vehicle (any lane)
    
            left(i)=1; 
            right(i)=1;
    
        elseif (ttc(i)<0 && rel_vel<0 && abs(ttc(i)) > t_min)    % target vehicle on the back of ego vehicle (ttc<0) (any lane)
            left(i) =1;
            right(i)=1;
    
        else 
            left(i) =0;
            right(i)=1;
    
        end

    % all actors on the right lane of the ego vehicle

    elseif actor_pos(2)-ego_pos(2) < 0
         
        if and(rel_vel>0, ttc(i) > t_min)  % target vehicles on the front of ego vehicle (any lane)
    
            left(i)=1;
            right(i)=1;
    
        elseif (ttc(i)<0 && rel_vel<0 && abs(ttc(i)) > t_min)    % target vehicle on the back of ego vehicle (ttc<0) (any lane)
            left(i) =1;
            right(i)=1;
    
        else 
            left(i) =1;
            right(i)=0;
    
        end
    end
%%

end

%% check if the vehicle is in the extreme end lanes

    if ego_pos(2)<y_lane(1) && ego_pos(2)>y_lane(2)

        LL=0; RL=1;
    elseif ego_pos(2) > y_lane(end) && ego_pos(2) < y_lane(end-1)
        RL=0; LL=1;
    else 

        RL=1;LL=1;
    end

%%
LL_avail = all(left) %&& LL;

RL_avail = all(right) %&& RL               %&& ~lcLeft ; this can be decided later 


%% final commands

stay = tend2stay || ~(tend2stay || LL_avail || RL_avail);
LL_Change =  ~tend2stay && LL_avail ;

RL_Change =  ~tend2stay && RL_avail && ~LL_Change ;
LCFlag = ~stay;
if LCFlag && LCinProgress
    LCFlag = false;
    stay = ~LCFlag;
end

%% 






end

== matlab function Candidacy_Exam_RR/Vehicle Dynamics/Info2ActorState/MATLAB Function2 ==
  data: aX input; Acceleration output; aY input; aZ input
function Acceleration = fcn(aX, aY, aZ)

Acceleration = [aX aY, aZ];

== matlab function Candidacy_Exam_RR/Vehicle Dynamics/Info2ActorState/MATLAB Function3 ==
  data: phiDot input; AngularVelocity output; thetaDot input; psiDot input
function AngularVelocity = fcn(phiDot, thetaDot, psiDot)

AngularVelocity = [phiDot thetaDot, psiDot];

== stateflow chart Candidacy_Exam_RR/Vehicle Dynamics/VehicleDynamics/engine-steer-brake dynamics/GearSelection1 ==
  state Park
    CurrGear = 0;
  state Reverse
    CurrGear = -1;
  state drive
    CurrGear = 1;
  (default) -> (junction 12)
  (junction 12) -> Reverse [order 3] : [DefaultGear == -1]
  (junction 12) -> drive [order 2] : [DefaultGear == 1]
  (junction 12) -> Park [order 1] : [DefaultGear == 0]
  (junction 12) -> Park [order 4] : %fallback to park
  drive -> Park [order 2] : [gear_cmd == 0 && allowShift(vc,Tbrake)]
  Park -> Reverse [order 2] : [gear_cmd == -1 && allowShift(vc,Tbrake)]
  Park -> drive [order 1] : [gear_cmd == 1 && allowShift(vc,Tbrake)]
  Reverse -> Park [order 2] : [gear_cmd == 0 && allowShift(vc,Tbrake)]
  drive -> Reverse [order 1] : [gear_cmd == -1 && allowShift(vc,Tbrake)]
  Reverse -> drive [order 1] : [gear_cmd == 1 && allowShift(vc,Tbrake)]
  data: Tdead parameter; Vdead parameter; vel function_input; brakeT function_input; allow function_output; CurrGear output; Tbrake input; vc input; gear_cmd input; DefaultGear parameter
  function allow = allowShift(vel, brakeT):
    | function allow = allowShift(vel, brakeT)
    | allow = (abs(vel) <= Vdead) && (abs(brakeT)>Tdead);
    | end

== matlab function Candidacy_Exam_RR/Vehicle Dynamics/VehicleDynamics/engine-steer-brake dynamics/compute net torque ==
  data: gear input; Tnet output; Tengine input; Tbrake input; vc input
function Tnet  = net_torque(gear,Tengine,Tbrake,vc)

%  --set engine torque based on current gear selection

if (gear == 0)
    %  --vehicle is in PARK, so force engine torque to zero
    Tengine = 0;
end

Tnet = Tengine + Tbrake*tanh(5*vc);

end

== matlab function Candidacy_Exam_RR/Vehicle Dynamics/VehicleDynamics/engine-steer-brake dynamics/gear selection state machine ==
  data: gear output; gear_cmd input; vc input; Tbrake input; Tdead input; Vdead input
function gear = gear_change_FSM(gear_cmd,vc,Tbrake,Tdead,Vdead)

persistent GEAR

%  The vehicle gear can take on one of the following enumerated values:
%  -1 = REVERSE
%   0 = PARK
%   1 = DRIVE

%  --initialize the local persistent variables

if isempty(GEAR)
    %  --default gear at startup is PARK
    %  Note:  Change this to 1 if you want car to initialize in DRIVE
    GEAR = 0;
end


%  --evaluate the gear change finite state machine

switch GEAR
    case 0  % vehicle is in PARK
        if (gear_cmd == 1)
            %  --check to see if we can shift to DRIVE
            if ((abs(vc) <= Vdead) && (abs(Tbrake) > Tdead))
                %  --shift to DRIVE
                GEAR = 1;
            end
            
        elseif (gear_cmd == 2)
            %  --check to see if we can shift to REVERSE
            if ((abs(vc) <= Vdead) && (abs(Tbrake) > Tdead))
                %  --shift to REVERSE
                GEAR = 2;
            end
        end
        
    case 1  % vehicle is in DRIVE
        if (gear_cmd == 0)
            %  --check to see if we can shift to PARK
            if ((abs(vc) <= Vdead) && (abs(Tbrake) > Tdead))
                %  --shift to PARK
                GEAR = 0;
            end
            
        elseif (gear_cmd == 2)
            %  --check to see if we can shift to REVERSE
            if ((abs(vc) <= Vdead) && (abs(Tbrake) > Tdead))
                %  --shift to REVERSE
                GEAR = 2;
            end
        end
        
    case -1  % vehicle is in REVERSE
        if (gear_cmd == 0)
            %  --check to see if we can shift to PARK
            if ((abs(vc) <= Vdead) && (abs(Tbrake) > Tdead))
                %  --shift to PARK
                GEAR = 0;
            end
            
        elseif (gear_cmd == 1)
            %  --check to see if we can shift to DRIVE
            if ((abs(vc) <= Vdead) && (abs(Tbrake) > Tdead))
                %  --shift to DRIVE
                GEAR = 1;
            end
        end
        
    otherwise  %  --should never be here
        if (vc > Vdead)
            %  --moving forward, so must be in DRIVE
            GEAR = 1;
        elseif (vc < -Vdead)
            %  --moving backward, so must be in REVERSE
            GEAR = 2;
        else
            %  --vehicle stoppped, so must be in PARK
            GEAR = 0;
        end

end


%  --output the current actual gear setting

gear = GEAR;

return

== matlab function Candidacy_Exam_RR/Behavioural Planner/MATLAB Function3 ==
  data: Dest input; D2D output; CurrentPose input
function D2D = fcn(Dest, CurrentPose)
%CurrentPose(2) = -CurrentPose(2);
%D2D = norm(Dest - CurrentPose(1:2)');
Dest = [Dest(2) Dest(1)]; 
CurrentPose = [CurrentPose(2) CurrentPose(1)];
D2D = norm(Dest - CurrentPose(1:2));
% D2D=sqrt((CurrentPose(1)-Dest(1,1))^2+(CurrentPose(2)-Dest(1,2))^2);
end
